simulink model "planeModel"  (R2019b)
settings: Solver=VariableStepAuto  StartTime=0.0  StopTime=10.0  RelTol=1e-3
values from neighbouring files (symbols this model uses):
  a_p1 = -A(3,3)    [Task2.m]
  a_p2 = A(3,5)    [Task2.m]
  d = deg2rad(1.5)    [Task2.m]
  k_dp = 500*k_dp1    (= 500)    [Task2.m]
settings Model: Creator=sendt  LastModifiedBy=sendt

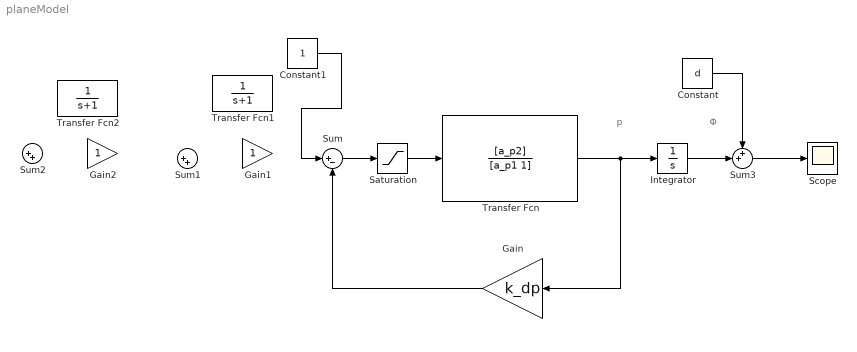
== system planeModel ==
  note: Φ
  note: p
  Constant : Constant  Value=d
  Constant1 : Constant
  Gain : Gain  Gain=k_dp
  Gain1 : Gain
  Gain2 : Gain
  Integrator : Integrator
  Saturation : Saturate  UpperLimit=deg2rad(30)  LowerLimit=deg2rad(-30)
  Scope : Scope
  Sum : Sum  Inputs=|+-
  Sum1 : Sum  Inputs=|++
  Sum2 : Sum  Inputs=|++
  Sum3 : Sum  Inputs=++|
  Transfer Fcn : TransferFcn  Numerator=[a_p2]  Denominator=[a_p1 1]
  Transfer Fcn1 : TransferFcn  Denominator=[1 1]
  Transfer Fcn2 : TransferFcn  Denominator=[1 1]
  wires:
  Gain/1 -> Sum/2
  Sum/1 -> Saturation/1
  Transfer Fcn/1 -> Gain/1, Integrator/1
  Integrator/1 -> Sum3/2
  Constant/1 -> Sum3/1
  Sum3/1 -> Scope/1
  Saturation/1 -> Transfer Fcn/1
  Constant1/1 -> Sum/1
